simulink model "RevisedStraightLine"  (R2015b)
settings: Solver=VariableStepAuto  StartTime=0.0  StopTime=1000  FixedStep=0.001  RelTol=1e-9
values from neighbouring files (symbols this model uses):
  a = [a1;a2;a3;a4]    [BeardMethod.m]    (also in RevisedMethod.m = 0)
  A = 3    [RevisedMethod.m]
  alpha = 1.65    [BeardMethod.m]    (also in OrbitCenter.m = abs((ang1-ang2)/2); RevisedMethod.m)
  ang = angle(i)    [BeardMethod.m]    (also in RevisedMethod.m = 0)
  b = [b1;b2;b3;b4]    [BeardMethod.m]    (also in RevisedMethod.m = 0)
  chi_inf = pi/2    (= 1.57079632679)    [BeardMethod.m]    (also in RevisedMethod.m)
  course_int = course_int+2*pi    (= 6.28318530718)    [BeardMethod.m]    (also in RevisedMethod.m = -0.785398163397)
  endx = E2(1)-6    [BeardMethod.m]    (also in RevisedMethod.m = 300)
  epsi = 0.1    [BeardMethod.m]    (also in RevisedMethod.m = 0.5)
  Gamma = 80    [RevisedMethod.m]
  i = 1    [BeardMethod.m]    (also in RevisedMethod.m = 1, go left, x decreases))
  k = 0.02    [BeardMethod.m]    (also in RevisedMethod.m = 0.1)
  kk = pi/2    (= 1.57079632679)    [BeardMethod.m]    (also in RevisedMethod.m)
  Method = 3    [RevisedMethod.m]
  phiA = pi    (= 3.14159265359)    [RevisedMethod.m]
  phiw = 230/180*pi    (= 4.01425727959)    [BeardMethod.m]    (also in RevisedMethod.m)
  Va = 13    [BeardMethod.m]    (also in RevisedMethod.m)
  Vg0 = sqrt((Va*sin(phi)+W*sin(phiw))^2+(Va*cos(phi)+W*cos(phiw))^2)    [InitialVg.m]    (also in RevisedMethod.m = InitialVg(A,0,W,phiw,Va,course_int))
  W = 6    [RevisedMethod.m]
  x_int = x.data(end)    [BeardMethod.m]    (also in RevisedMethod.m = 0)
  y_int = y.data(end)    [BeardMethod.m]    (also in RevisedMethod.m = 80)
libraries: simulink x1
settings Model: Creator=Bingyu Zhou  LastModifiedBy=Bingyu Zhou

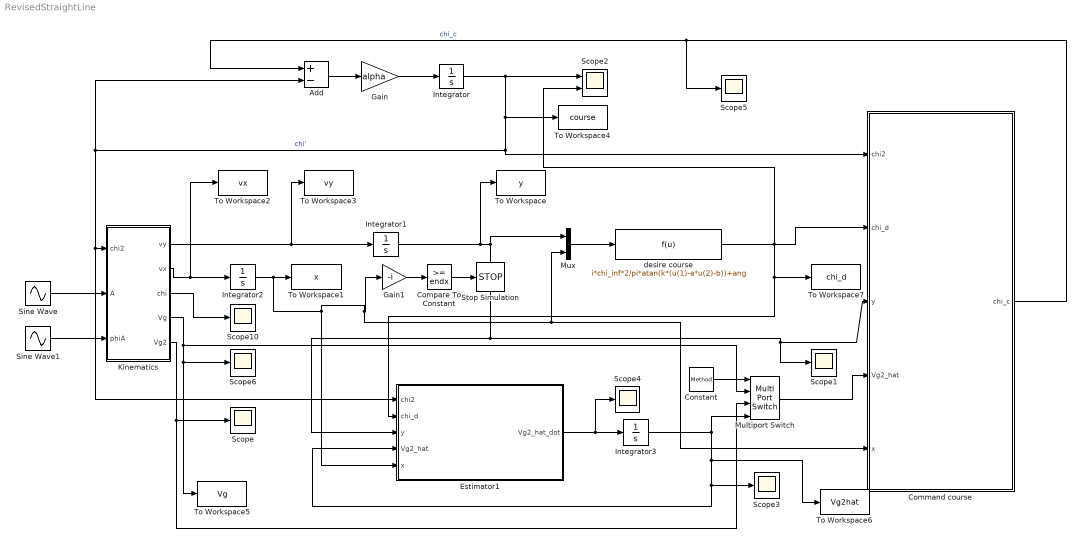
== system RevisedStraightLine ==
  Add : Sum  Inputs=+-
  Command course : Subsystem
  Compare To Constant : simulink/Logic and Bit Operations/Compare To Constant  relop=>=  const=endx  OutDataTypeStr=boolean
  Constant : Constant  Value=Method
  Estimator1 : MATLAB Function  TreatAsAtomicUnit=on
  Gain : Gain  Gain=alpha
  Gain1 : Gain  Gain=-i
  Integrator : Integrator  InitialCondition=course_int
  Integrator1 : Integrator  InitialCondition=y_int
  Integrator2 : Integrator  InitialCondition=x_int
  Integrator3 : Integrator  InitialCondition=Vg0
  Kinematics : Subsystem
  Multiport Switch : MultiPortSwitch
  Mux : Mux  Inputs=2
  Scope{,1,3..6,10} (7 alike) : Scope
  Scope2 : Scope  NumInputPorts=2
  Sine Wave : Sin  Amplitude=A  Frequency=0.1  Phase=pi/2  SampleTime=0
  Sine Wave1 : Sin  Amplitude=phiA  Frequency=0.1  SampleTime=0
  Stop Simulation : Stop
  To Workspace : ToWorkspace  VariableName=y  SaveFormat=Timeseries  SampleTime=-1
  To Workspace1 : ToWorkspace  VariableName=x  SaveFormat=Timeseries  SampleTime=-1
  To Workspace2 : ToWorkspace  VariableName=vx  SaveFormat=Timeseries  SampleTime=-1
  To Workspace3 : ToWorkspace  VariableName=vy  SaveFormat=Timeseries  SampleTime=-1
  To Workspace4 : ToWorkspace  VariableName=course  SaveFormat=Timeseries  SampleTime=-1
  To Workspace5 : ToWorkspace  VariableName=Vg  SaveFormat=Timeseries  SampleTime=-1
  To Workspace6 : ToWorkspace  VariableName=Vg2hat  SaveFormat=Timeseries  SampleTime=-1
  To Workspace7 : ToWorkspace  VariableName=chi_d  SaveFormat=Timeseries  SampleTime=-1
  desire course : Fcn  Expr=i*chi_inf*2/pi*atan(k*(u(1)-a*u(2)-b))+ang
  wires:
  Add/1 -> Gain/1
  Gain/1 -> Integrator/1
  Integrator/1 -> Scope2/1, To Workspace4/1, Command course/1(chi2), Add/2, Estimator1/1(chi2), Kinematics/1(chi2)  "chi'"
  Integrator1/1 -> To Workspace/1, Estimator1/3(y), Scope1/1, Command course/3(y), Mux/1
  Command course/1(chi_c) -> Scope5/1, Add/1  "chi_c"
  Integrator2/1 -> Estimator1/5(x), Command course/5(x), Mux/2, Gain1/1, To Workspace1/1
  Estimator1/1(Vg2_hat_dot) -> Scope4/1, Integrator3/1
  Integrator3/1 -> Scope3/1, Estimator1/4(Vg2_hat), To Workspace6/1, Multiport Switch/4
  Kinematics/1(vy) -> Integrator1/1, To Workspace3/1
  Kinematics/2(vx) -> To Workspace2/1, Integrator2/1
  Kinematics/3(chi) -> Scope10/1
  Kinematics/4(Vg) -> Multiport Switch/2, To Workspace5/1, Scope6/1
  Compare To Constant/1 -> Stop Simulation/1
  Gain1/1 -> Compare To Constant/1
  Kinematics/5(Vg2) -> Multiport Switch/3, Scope/1
  Sine Wave1/1 -> Kinematics/3(phiA)
  Sine Wave/1 -> Kinematics/2(A)
  Mux/1 -> desire course/1
  desire course/1 -> Scope2/2, Estimator1/2(chi_d), To Workspace7/1, Command course/2(chi_d)
  Constant/1 -> Multiport Switch/1
  Multiport Switch/1 -> Command course/4(Vg2_hat)

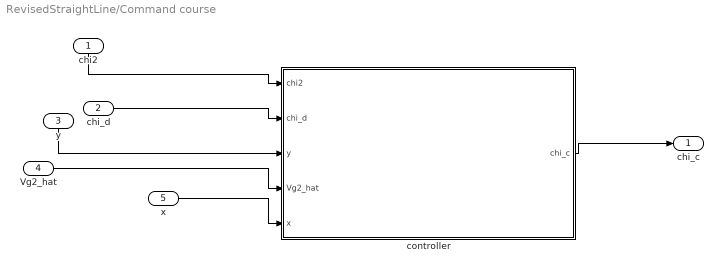
== system RevisedStraightLine/Command course ==
  chi2 : Inport
  chi_d : Inport  Port=2
  y : Inport  Port=3
  Vg2_hat : Inport  Port=4
  x : Inport  Port=5
  controller : MATLAB Function  TreatAsAtomicUnit=on
  chi_c : Outport
  wires:
  chi_d/1 -> controller/2(chi_d)
  controller/1(chi_c) -> chi_c/1
  chi2/1 -> controller/1(chi2)
  y/1 -> controller/3(y)
  Vg2_hat/1 -> controller/4(Vg2_hat)
  x/1 -> controller/5(x)

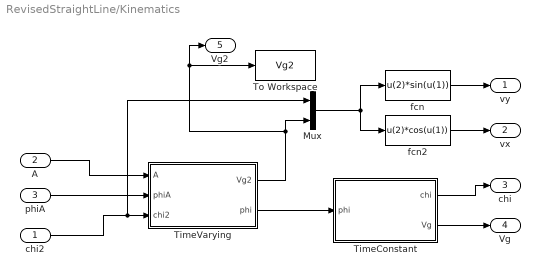
== system RevisedStraightLine/Kinematics ==
  chi2 : Inport
  A : Inport  Port=2
  phiA : Inport  Port=3
  Mux : Mux  Inputs=2
  TimeConstant : MATLAB Function  TreatAsAtomicUnit=on
  TimeVarying : MATLAB Function  TreatAsAtomicUnit=on
  To Workspace : ToWorkspace  VariableName=Vg2  SaveFormat=Timeseries  SampleTime=-1
  fcn : Fcn  Expr=u(2)*sin(u(1))
  fcn2 : Fcn  Expr=u(2)*cos(u(1))
  vy : Outport
  vx : Outport  Port=2
  chi : Outport  Port=3
  Vg : Outport  Port=4
  Vg2 : Outport  Port=5
  wires:
  A/1 -> TimeVarying/1(A)
  fcn/1 -> vy/1
  Mux/1 -> fcn/1, fcn2/1
  fcn2/1 -> vx/1
  TimeVarying/2(phi) -> TimeConstant/1(phi)
  TimeConstant/2(Vg) -> Vg/1
  phiA/1 -> TimeVarying/2(phiA)
  TimeVarying/1(Vg2) -> Vg2/1, To Workspace/1, Mux/2
  TimeConstant/1(chi) -> chi/1
  chi2/1 -> Mux/1, TimeVarying/3(chi2)

== matlab function RevisedStraightLine/Kinematics/TimeVarying ==
  data: A input; phiA input; W parameter; phiw parameter; chi2 input; Va parameter; Vg2 output; phi output
function [Vg2,phi] = TimeVarying(A,phiA,W,phiw,chi2,Va)
% calculate the Vg' and heading angle(phi)

%calculate the whole current vector including constant current (W,phiw) and time
%varying current(A,phiA)
% C cos(phic) = W cos(phiw)+ A cos(phiA)
% C sin(phic) = W sin(phiw)+ A sin(phiA)
phic = atan2(W*sin(phiw)+A*sin(phiA),W*cos(phiw)+A*cos(phiA));
C = sqrt((W*sin(phiw)+A*sin(phiA))^2+(W*cos(phiw)+A*cos(phiA))^2);

%Calculate Vg' and phi based on Va and C
%Vg' cos(X') = Va cos(phi) + C cos(phic)
%Vg' sin(X') = Va sin(phi) + C sin(phic)
Vg2 = C*cos(phic-chi2)+sqrt(Va^2-C^2*sin(phic-chi2)^2);
phi = atan2(-C/Va*sin(phic-chi2),sqrt(1-C^2/Va^2*sin(phic-chi2)^2))+chi2; %heading angle
end

== matlab function RevisedStraightLine/Command course/controller ==
  data: chi2 input; chi_d input; y input; Vg2_hat input; chi_c output; epsi parameter; chi_inf parameter; k parameter; kk parameter; alpha parameter; i parameter; x input; a parameter; b parameter
function chi_c = CommandCourse(chi2,chi_d,y,Vg2_hat,epsi,chi_inf,k,kk,alpha,i,x,a,b)
%generate command course angle chi_c
term =(chi2-chi_d)/epsi;
if abs(term)<=1
    sat=term;
else
    sat=sign(term);
end

e = y-(a*x+b);
chi_c=chi2+i*chi_inf*2/pi/alpha*(k*(sin(chi2)-a*cos(chi2)))/(1+(k*(e))^2)*(Vg2_hat)-kk/alpha*sat;


end

== matlab function RevisedStraightLine/Kinematics/TimeConstant ==
  data: phi input; chi output; Va parameter; W parameter; phiw parameter; Vg output
function [chi,Vg] = TimeConstant(phi,Va,W,phiw)
%calculation of Vg and chi

chi = atan2(Va*sin(phi)+W*sin(phiw),Va*cos(phi)+W*cos(phiw));
Vg = sqrt((Va*sin(phi)+W*sin(phiw))^2+(Va*cos(phi)+W*cos(phiw))^2);

end

== matlab function RevisedStraightLine/Estimator1 ==
  data: chi2 input; chi_d input; y input; Vg2_hat input; Vg2_hat_dot output; y_int parameter; W parameter; Va parameter; epsi parameter; phiw parameter; chi_inf parameter; k parameter; kk parameter; i parameter; a parameter; b parameter; x input; Gamma parameter
function Vg2_hat_dot = estimator(chi2,chi_d,y,Vg2_hat,y_int,W,Va,epsi,phiw,chi_inf,k,kk,i,a,b,x,Gamma)
%estimator of Vg'

rho = y_int^2/pi^2; %positive scale factor used to weight the terms so that y and chi are similar in magnitude

diff_chi = chi2-chi_d; % error of course angle

term =diff_chi/epsi;
if abs(term)<=1
    sat=term;
else
    sat=sign(term);
end
% derivative of Vg' over x'
der = W*sin(phiw-chi2)+(Va^2-W^2*(sin(phiw-chi2))^2)^(-0.5)*W^2*sin(phiw-chi2)*cos(phiw-chi2); % partial derivative of Vg' over chi'

e = y-(a*x+b);

Vg2_hat_dot =-i*Gamma*rho*diff_chi*chi_inf*2/pi*(k*(sin(chi2)-a*cos(chi2)))/(1+(k*(e))^2)+der*(i*chi_inf*2/pi*(k*(sin(chi2)-a*cos(chi2)))/(1+(k*(e))^2)*Vg2_hat-kk*sat);

end
